simulink model "Aufgabe3_Simulink"  (R2025b)
settings: Solver=VariableStepAuto  StartTime=0.0  StopTime=10.0  RelTol=1e-3
undefined symbols (not defined in the file): A, B, C, D, delta_sim
settings Model: Creator=elias  LastModifiedBy=elias

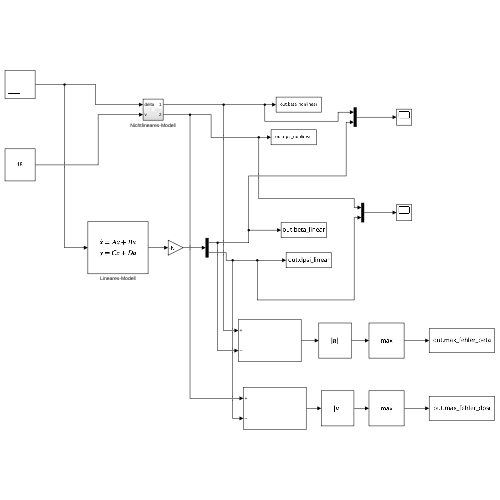
[thumbnail: Simulink's stored preview of the top-level diagram]
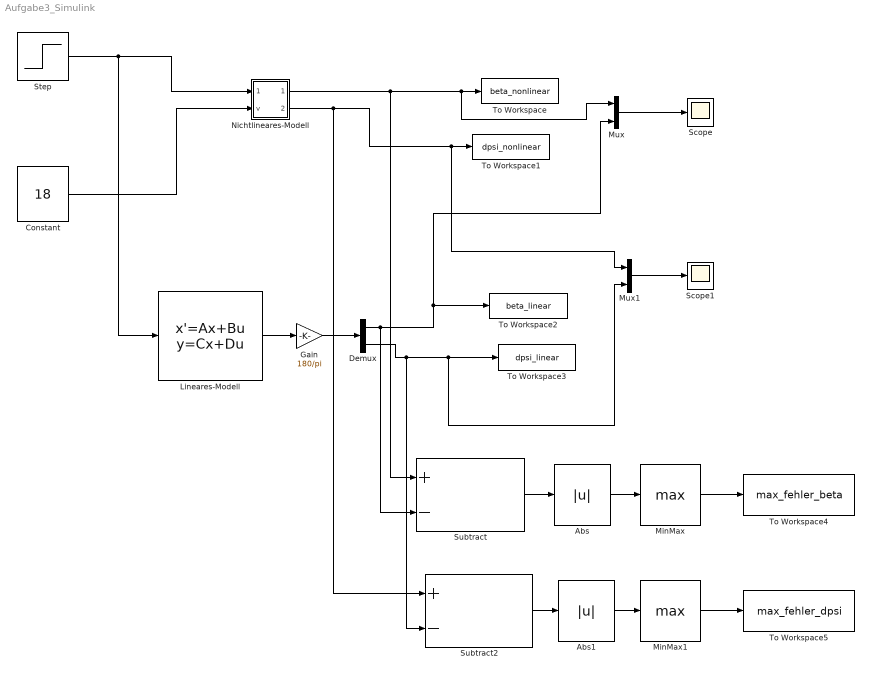
== system Aufgabe3_Simulink ==
  Abs : Abs  SaturateOnIntegerOverflow=off
  Abs1 : Abs  SaturateOnIntegerOverflow=off
  Constant : Constant  Value=18
  Demux : Demux  Outputs=2
  Gain : Gain  Gain=180/pi
  Lineares-Modell : StateSpace  A=A  B=B  C=C  D=D  InitialCondition=0
  MinMax : MinMax  Function=max
  MinMax1 : MinMax  Function=max
  Mux : Mux  Inputs=2
  Mux1 : Mux  Inputs=2
  Nichtlineares-Modell : Subsystem
  Scope : Scope
      settings: ActiveDisplayYMinimum=-1.0999906234404921  ActiveDisplayYMaximum=0.36221552661549006
  Scope1 : Scope
      settings: ActiveDisplayYMinimum=-15.253412733311251  ActiveDisplayYMaximum=62.000879060715192
  Step : Step  Time=0  After=delta_sim  SampleTime=0
  Subtract : Sum  Inputs=+-
  Subtract2 : Sum  Inputs=+-
  To Workspace : ToWorkspace  VariableName=beta_nonlinear  SaveFormat=Timeseries  SampleTime=-1
  To Workspace1 : ToWorkspace  VariableName=dpsi_nonlinear  SaveFormat=Timeseries  SampleTime=-1
  To Workspace2 : ToWorkspace  VariableName=beta_linear  SaveFormat=Timeseries  SampleTime=-1
  To Workspace3 : ToWorkspace  VariableName=dpsi_linear  SaveFormat=Timeseries  SampleTime=-1
  To Workspace4 : ToWorkspace  VariableName=max_fehler_beta  SampleTime=-1
      settings: Save2DSignal=2-D array (concatenate along first dimension)
  To Workspace5 : ToWorkspace  VariableName=max_fehler_dpsi  SampleTime=-1
      settings: Save2DSignal=2-D array (concatenate along first dimension)
  wires:
  Nichtlineares-Modell/1(Out1) -> Subtract/1, Mux/1, To Workspace/1
  Nichtlineares-Modell/2(Out2) -> Subtract2/1, Mux1/1, To Workspace1/1
  Step/1 -> Lineares-Modell/1, Nichtlineares-Modell/1(delta)
  Constant/1 -> Nichtlineares-Modell/2(v)
  Demux/1 -> Mux/2, To Workspace2/1, Subtract/2
  Demux/2 -> Subtract2/2, Mux1/2, To Workspace3/1
  Mux/1 -> Scope/1
  Mux1/1 -> Scope1/1
  Lineares-Modell/1 -> Gain/1
  Gain/1 -> Demux/1
  Subtract/1 -> Abs/1
  Abs/1 -> MinMax/1
  MinMax/1 -> To Workspace4/1
  Abs1/1 -> MinMax1/1
  Subtract2/1 -> Abs1/1
  MinMax1/1 -> To Workspace5/1

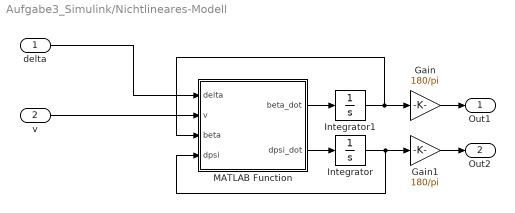
== system Aufgabe3_Simulink/Nichtlineares-Modell ==
  delta : Inport
  v : Inport  Port=2
  Gain : Gain  Gain=180/pi
  Gain1 : Gain  Gain=180/pi
  Integrator : Integrator
  Integrator1 : Integrator
  MATLAB Function : MATLAB Function  TreatAsAtomicUnit=on
  Out1 : Outport
  Out2 : Outport  Port=2
  wires:
  Integrator/1 -> Gain1/1, MATLAB Function/4(dpsi)
  MATLAB Function/2(dpsi_dot) -> Integrator/1
  Integrator1/1 -> Gain/1, MATLAB Function/3(beta)
  Gain/1 -> Out1/1
  delta/1 -> MATLAB Function/1(delta)
  v/1 -> MATLAB Function/2(v)
  MATLAB Function/1(beta_dot) -> Integrator1/1
  Gain1/1 -> Out2/1

== matlab function Aufgabe3_Simulink/Nichtlineares-Modell/MATLAB Function ==
  data: delta input; beta_dot output; v input; beta input; dpsi input; dpsi_dot output; p parameter
function [beta_dot, dpsi_dot] = fcn(delta, v, beta, dpsi, p)

cb = cos(beta);

% 1. Schräglaufwinkel berechnen (mit Parametern aus dem Struct p)
    alpha_v = delta - (p.lf * dpsi) / (v * cb) + tan(beta);
    alpha_h = (p.lr * dpsi) / (v * cb) - tan(beta);

    % Reifen-Seitenkräfte (wie in deinem Skript)
    Fy_v = p.cf * alpha_v;
    Fy_h = p.cr * alpha_h;

    % 2. Differentialgleichungen (Zustandsableitungen)
    beta_dot = -dpsi + (1 / (p.m * v)) * ((Fy_v * cos(delta) / cb) + (Fy_h / cb));
    dpsi_dot = (1 / p.Jz) * (p.lf * Fy_v * cos(delta) - p.lr * Fy_h);

end
